simulink model "VerifyTrimPoint_model"  (R2018b)
settings: Solver=VariableStepAuto  StartTime=0.0  StopTime=tFinal  RelTol=1e-3
values from neighbouring files (symbols this model uses):
  Uo = [Inputs(1).u ... (first row only)    [ExtractTrimPoint.m]
undefined symbols (not defined in the file or in its folder): GEOMETRY
libraries: PlanarVehicle x2
settings Model: Creator=Christopher  LastModifiedBy=Christopher
settings DataIOCC: ExternalInput=getinputstruct(op_trim11)  InitialState=getstatestruct(op_trim11)

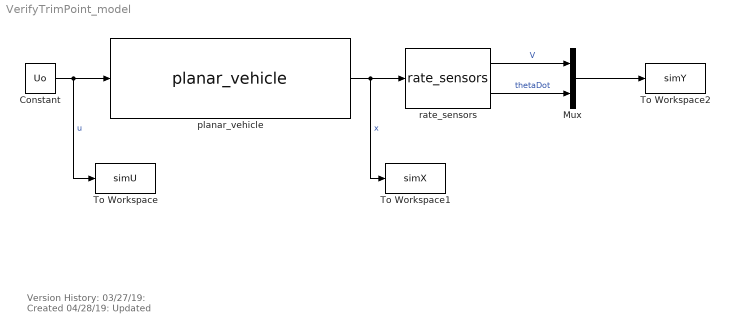
== system VerifyTrimPoint_model ==
  note: Version History:
      | 03/27/19: Created
      | 04/28/19: Updated
  Constant : Constant  Value=Uo
  Mux : Mux  Inputs=2
  To Workspace : ToWorkspace  VariableName=simU  SaveFormat=Timeseries  SampleTime=-1
  To Workspace1 : ToWorkspace  VariableName=simX  SaveFormat=Timeseries  SampleTime=-1
  To Workspace2 : ToWorkspace  VariableName=simY  SaveFormat=Timeseries  SampleTime=-1
  planar_vehicle : PlanarVehicle/planar_vehicle  m=GEOMETRY.mass  Ib=GEOMETRY.Ib  Fmax=PROPULSION.Fmax  Mmax=PROPULSION.Mmax  x0=SIMULATION.X_0  CT=ENVIRONMENT.CT  CR=ENVIRONMENT.CR
  rate_sensors : PlanarVehicle/rate_sensors
  wires:
  Constant/1 -> To Workspace/1, planar_vehicle/1  "u"
  planar_vehicle/1 -> rate_sensors/1, To Workspace1/1  "x"
  rate_sensors/1 -> Mux/1  "V"
  rate_sensors/2 -> Mux/2  "thetaDot"
  Mux/1 -> To Workspace2/1
